simulink model "project_2023_12_18_P114"  (R2017b)
settings: Solver=ode5  StartTime=0.0  StopTime=100  FixedStep=0.01  RelTol=1e-3
undefined symbols (not defined in the file): k
libraries: simulink x1
settings Model: Creator=Administrator  LastModifiedBy=Administrator

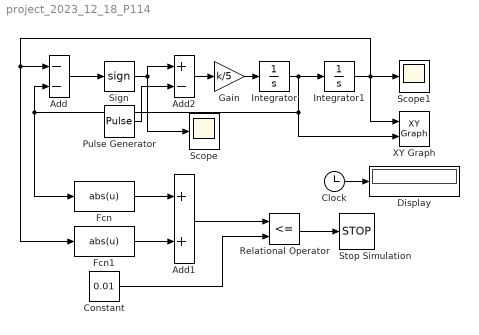
== system project_2023_12_18_P114 ==
  Add : Sum  Inputs=--
  Add1 : Sum
  Add2 : Sum  Inputs=+-
  Clock : Clock
  Constant : Constant  Value=0.01
  Display : Display
  Fcn : Fcn  Expr=abs(u)
  Fcn1 : Fcn  Expr=abs(u)
  Gain : Gain  Gain=k/5
  Integrator : Integrator
  Integrator1 : Integrator  InitialCondition=12
  Pulse Generator : DiscretePulseGenerator  PulseType=Time based  Amplitude=10  Period=1
  Relational Operator : RelationalOperator  Operator=<=  OutDataTypeStr=boolean  RndMeth=Simplest
  Scope : Scope
  Scope1 : Scope
  Sign : Signum  ZeroCross=off
  Stop Simulation : Stop
  XY Graph : simulink/Sinks/XY Graph  xmin=-1  xmax=1  ymin=-1  ymax=1  st=-1
  wires:
  Add/1 -> Sign/1
  Sign/1 -> Add2/1, Scope/1
  Integrator/1 -> XY Graph/2, Fcn/1, Add/2, Integrator1/1
  Integrator1/1 -> XY Graph/1, Add/1, Fcn1/1, Scope1/1
  Fcn/1 -> Add1/1
  Fcn1/1 -> Add1/2
  Add1/1 -> Relational Operator/1
  Constant/1 -> Relational Operator/2
  Clock/1 -> Display/1
  Relational Operator/1 -> Stop Simulation/1
  Gain/1 -> Integrator/1
  Add2/1 -> Gain/1
  Pulse Generator/1 -> Add2/2
